simulink model "ms_estimate__SG_"  (R2020a)
settings: Solver=FixedStepDiscrete  StartTime=0.0  StopTime=tf  RelTol=1e-3  EnableMultiTasking=on
PreLoadFcn:
  | Ts = 0.001;
  | FPGA_Frequency = 75000000;
InitFcn:
  | Ts = 0.001;
  | FPGA_Frequency = 75000000;
values from neighbouring files (symbols this model uses):
  A = 0.5    [ms_estimate__main.m]
  ts = 1/fs    (= 0.0001)    [ms_estimate__main.m]
libraries: dspfdesign x4, slrtlib x2, dspsrcs4 x1, SG_library x1
settings Model: SimulationMode=external  Creator=lab  LastModifiedBy=padlewsk
settings SolverCC: ConcurrentTasks=on  AutoInsertRateTranBlk=on  InsertRTBMode=Never (minimum delay)
settings DataIOCC: LimitDataPoints=on  SaveFormat=StructureWithTime  SaveOutput=off  SignalLogging=off  DSMLogging=off  SaveTime=off  ReturnWorkspaceOutputs=off
settings OptimizationCC: BlockReduction=off  OptimizeBlockIOStorage=off  BufferReuse=off  GlobalBufferReuse=off  ExpressionFolding=off  LocalBlockOutputs=off  OptimizeDataStoreBuffers=off  BusAssignmentInplaceUpdate=off
settings DebuggingCC: UnconnectedInputMsg=none  UnconnectedOutputMsg=none  UnconnectedLineMsg=none
settings HardwareCC: ProdBitPerPointer=32  ProdBitPerSizeT=32  ProdBitPerPtrDiffT=32  ProdLargestAtomicFloat=None  ProdWordSize=32  ProdLongLongMode=on  ProdHWDeviceType=Generic->32-bit x86 compatible
settings SFSimCC: CustomCodeUndefinedFunction=UseInterfaceOnly
settings RTWCC: Description=Simulink Real-Time  SystemTargetFile=slrt.tlc  TemplateMakefile=slrt_default_tmf  CodeExecutionProfiling=on  RTWCompilerOptimization=on
settings SimulinkRealTimeCC: SupportVariableSizeSignals=on  xPCConcurrentTasks=on

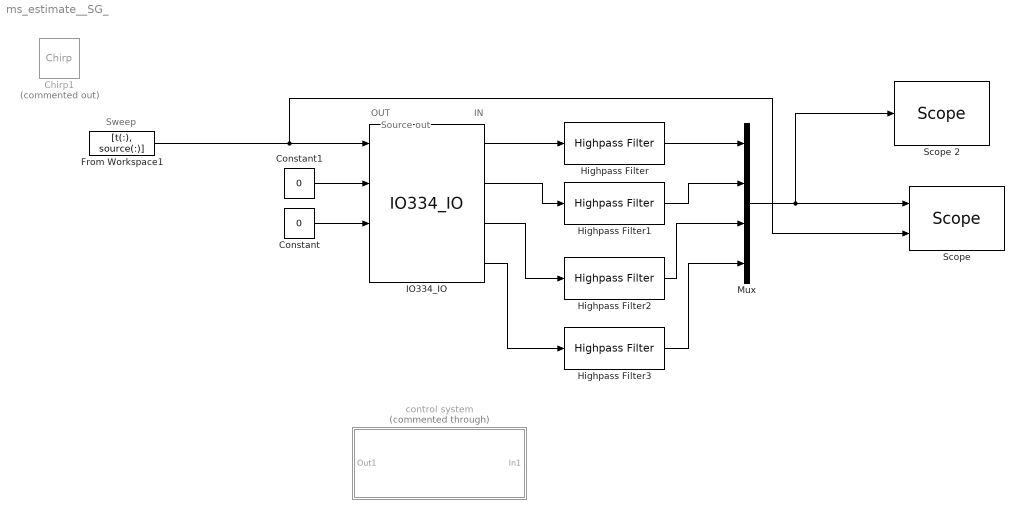
== system ms_estimate__SG_ ==
  note: OUT
  note: Sweep
  note: Source out
  note: IN
  Chirp1 : dspsrcs4/Chirp  Commented=on  sweep=Linear  mode=Bidirectional  f0=80  f1=1100  t1=0  Tsweep=10  phase=0  Ts=2.5e-05  spf=1  datatype=Double  OutputFrames=off
  Constant : Constant  Value=0  SampleTime=ts
  Constant1 : Constant  Value=0  SampleTime=ts
  From Workspace1 : FromWorkspace  VariableName=[t(:), source(:)]  SampleTime=ts  OutputAfterFinalValue=Setting to zero
  Highpass Filter : dspfdesign/Highpass Filter  FilterType=IIR  DesignForMinimumOrder=off  FilterOrder=4  StopbandFrequency=8e3  PassbandFrequency=5  StopbandAttenuation=80  PassbandRipple=0.1  InheritSampleRate=off  SampleRate=40000  SimulateUsing=Interpreted execution  roundingMode=Floor  coeffsDataTypeStr=fixdt(1,16)
  Highpass Filter1 : dspfdesign/Highpass Filter  FilterType=IIR  DesignForMinimumOrder=off  FilterOrder=4  StopbandFrequency=8e3  PassbandFrequency=5  StopbandAttenuation=80  PassbandRipple=0.1  InheritSampleRate=off  SampleRate=40000  SimulateUsing=Interpreted execution  roundingMode=Floor  coeffsDataTypeStr=fixdt(1,16)
  Highpass Filter2 : dspfdesign/Highpass Filter  FilterType=IIR  DesignForMinimumOrder=off  FilterOrder=4  StopbandFrequency=8e3  PassbandFrequency=5  StopbandAttenuation=80  PassbandRipple=0.1  InheritSampleRate=off  SampleRate=40000  SimulateUsing=Interpreted execution  roundingMode=Floor  coeffsDataTypeStr=fixdt(1,16)
  Highpass Filter3 : dspfdesign/Highpass Filter  FilterType=IIR  DesignForMinimumOrder=on  FilterOrder=50  StopbandFrequency=4  PassbandFrequency=5  StopbandAttenuation=80  PassbandRipple=0.1  InheritSampleRate=off  SampleRate=40000  SimulateUsing=Interpreted execution  roundingMode=Floor  coeffsDataTypeStr=fixdt(1,16)
  IO334_IO : SG_library/Built elements/IO334_IO
      settings: SourceProductName=Custom Speedgoat implementations
  Mux : Mux
  "Scope " : slrtlib/Displays and Logging/Scope   scopeno=2  scopetype=Host  autostart=on  viewmode=Graphical redraw  formatstr='%15.6f'  grid=on  ylimits=[0,0]  nosamples=fs  noprepostsamples=0  interleave=tf  triggermode=Signal triggering  triggersignal=1  trigsignalfromport=on  triggerlevel=A - A/10  triggerslope=Either  triggerscope=1  triggersample=0  filename=data.dat  mode=Lazy  writesize=512  autorestart=off  dynamicfilemode=off  maxwritefilesize=512*1024^2
  Scope 2 : slrtlib/Displays and Logging/Scope   scopeno=1  scopetype=Target  autostart=on  viewmode=Graphical redraw  formatstr='%15.6f'  grid=on  ylimits=[-10,10]  nosamples=1/ts  noprepostsamples=0  interleave=1  triggermode=FreeRun  triggersignal=1  trigsignalfromport=off  triggerlevel=0.0  triggerslope=Either  triggerscope=1  triggersample=0  filename=data.dat  mode=Lazy  writesize=512  autorestart=off  dynamicfilemode=off  maxwritefilesize=512*1024^2
  control system : Subsystem  Commented=through
  wires:
  IO334_IO/1 -> Highpass Filter/1
  IO334_IO/2 -> Highpass Filter1/1
  IO334_IO/3 -> Highpass Filter2/1
  IO334_IO/4 -> Highpass Filter3/1
  Constant1/1 -> IO334_IO/2
  Highpass Filter/1 -> Mux/1
  Highpass Filter1/1 -> Mux/2
  Highpass Filter2/1 -> Mux/3
  Highpass Filter3/1 -> Mux/4
  Constant/1 -> IO334_IO/3
  Mux/1 -> Scope 2/1, "Scope "/1
  From Workspace1/1 -> "Scope "/2, IO334_IO/1

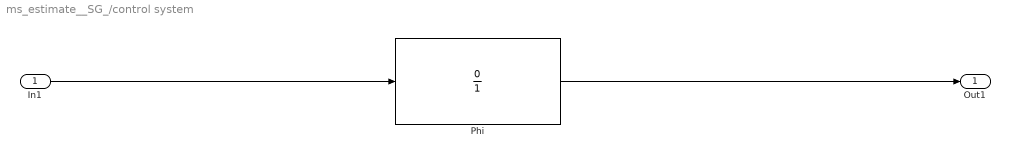
== system ms_estimate__SG_/control system ==
  In1 : Inport
  Phi : DiscreteTransferFcn  Numerator=[0]  Denominator=[1]
  Out1 : Outport
  wires:
  In1/1 -> Phi/1
  Phi/1 -> Out1/1
